simulink model "sim_sys_robot"  (R2017a)
settings: Solver=VariableStepAuto  StartTime=0.0  StopTime=1  MaxStep=0.01  RelTol=1e-4  EnableMultiTasking=on
values from neighbouring files (symbols this model uses):
  n_juncoes = size(vars, 1)    [animation.m]    (also in puma.m = 4; scara.m = 4)
libraries: simulink x1
settings Model: Creator=julio  LastModifiedBy=julio
settings DataIOCC: LimitDataPoints=on  SaveOutput=off  SaveTime=off
settings OptimizationCC: ExpressionDepthLimit=2147483647  LifeSpan=1
settings DebuggingCC: AlgebraicLoopMsg=none  UnderspecifiedInitializationDetection=Classic  MergeDetectMultiDrivingBlocksExec=none  FcnCallInpInsideContextMsg=warning  AllowSymbolicDim=off  StateNameClashWarn=warning  SFUnexpectedBacktrackingDiag=warning  SFNoUnconditionalDefaultTransitionDiag=warning  SFExecutionAtInitializationDiag=none
settings GRTTargetCC: TargetLangStandard=C89/C90 (ANSI)  GeneratePreprocessorConditionals=Disable all  CombineOutputUpdateFcns=off  GRTInterface=on

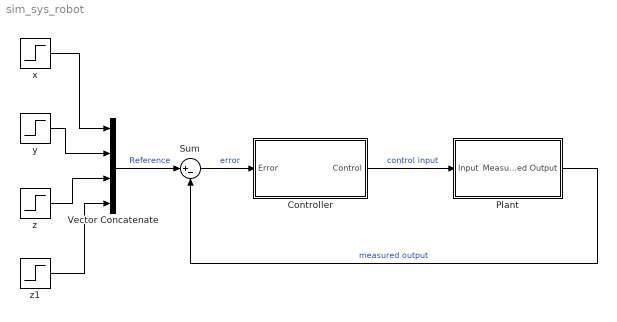
== system sim_sys_robot ==
  Controller : Subsystem
  Plant : Subsystem
  Sum : Sum  Inputs=|+-
  Vector Concatenate : Concatenate  NumInputs=4
  x : Step  After=0  SampleTime=0
  y : Step  After=0  SampleTime=0
  z : Step  After=0  SampleTime=0
  z1 : Step  After=0  SampleTime=0
  wires:
  Plant/1(Measured Output) -> Sum/2  "measured output"
  Sum/1 -> Controller/1(Error)  "error"
  Controller/1(Control) -> Plant/1(Input)  "control input"
  Vector Concatenate/1 -> Sum/1  "Reference"
  y/1 -> Vector Concatenate/2
  z/1 -> Vector Concatenate/3
  x/1 -> Vector Concatenate/1
  z1/1 -> Vector Concatenate/4

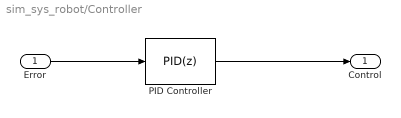
== system sim_sys_robot/Controller ==
  Error : Inport  PortDimensions=n_juncoes
  PID Controller : simulink/Continuous/PID Controller  Controller=PID  TimeDomain=Discrete-time  SampleTime=0.1  IntegratorMethod=Forward Euler  FilterMethod=Forward Euler  Form=Parallel  UseFilter=on  ControllerParametersSource=internal  P=1.2  I=22  D=0.02  N=20  InitialConditionSource=internal  InitialConditionForIntegrator=0  InitialConditionForFilter=0  ExternalReset=none  LimitOutput=off  UpperSaturationLimit=inf  LowerSaturationLimit=-inf  LinearizeAsGain=on  AntiWindupMode=none  Kb=1  TrackingMode=off  Kt=1  PParamMin=[]  PParamMax=[]  IParamMin=[]  IParamMax=[]  DParamMin=[]  DParamMax=[]  NParamMin=[]  NParamMax=[]  KbParamMin=[]  KbParamMax=[]  KtParamMin=[]  KtParamMax=[]  POutMin=[]  POutMax=[]  IOutMin=[]  IOutMax=[]  DOutMin=[]  DOutMax=[]  NOutMin=[]  NOutMax=[]  KbOutMin=[]  KbOutMax=[]  KtOutMin=[]  KtOutMax=[]  IntegratorOutMin=[]  IntegratorOutMax=[]  FilterOutMin=[]  FilterOutMax=[]  SumOutMin=[]  SumOutMax=[]  SumI1OutMin=[]  SumI1OutMax=[]  SumI2OutMin=[]  SumI2OutMax=[]  SumI3OutMin=[]  SumI3OutMax=[]  SumDOutMin=[]  SumDOutMax=[]  SaturationOutMin=[]  SaturationOutMax=[]  IntegratorContinuousStateAttributes=''  IntegratorStateMustResolveToSignalObject=off  IntegratorRTWStateStorageClass=Auto  FilterContinuousStateAttributes=''  FilterStateMustResolveToSignalObject=off  FilterRTWStateStorageClass=Auto  DifferentiatorICPrevScaledInput=0  DifferentiatorOutMin=[]  DifferentiatorOutMax=[]  InitialConditionSetting=State (most efficient)
  Control : Outport  PortDimensions=n_juncoes
  wires:
  Error/1 -> PID Controller/1
  PID Controller/1 -> Control/1

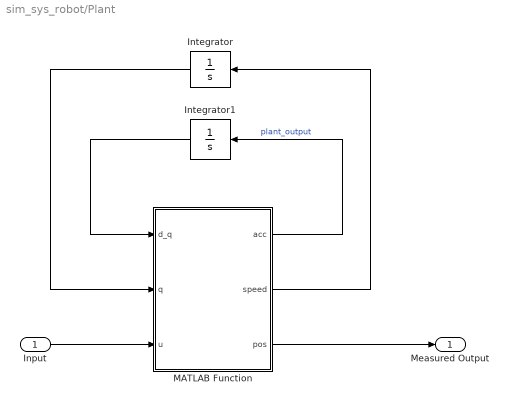
== system sim_sys_robot/Plant ==
  Input : Inport  PortDimensions=n_juncoes
  Integrator : Integrator  InitialCondition=zeros(n_juncoes, 1)
  Integrator1 : Integrator  InitialCondition=zeros(n_juncoes, 1)
  MATLAB Function : MATLAB Function  TreatAsAtomicUnit=on
  Measured Output : Outport  PortDimensions=n_juncoes
  wires:
  Input/1 -> MATLAB Function/3(u)
  MATLAB Function/2(speed) -> Integrator/1
  Integrator/1 -> MATLAB Function/2(q)
  MATLAB Function/1(acc) -> Integrator1/1  "plant_output"
  Integrator1/1 -> MATLAB Function/1(d_q)
  MATLAB Function/3(pos) -> Measured Output/1

== matlab function sim_sys_robot/Plant/MATLAB Function ==
  data: d_q input; acc output; q input; speed output; u input size=n_juncoes; pos output
function [acc, speed, pos] = system(d_q, q, u)

    [m, n] = size(q);
    coder.extrinsic('get_matrices');
    
    D = eye(m);
    C = zeros(m, m);
    g = zeros(m, 1);
    
    [D, C, g] = get_matrices(d_q, q);
    
    acc = inv(D)*(u-C*d_q-g);
    speed = d_q;
    pos = q;
end
